simulink model "balance_leg_sl"  (R2022b)
settings: Solver=VariableStepAuto  StartTime=0.0  StopTime=10  RelTol=1e-3
values from neighbouring files (symbols this model uses):
  K = get_K_from_LQR(R_w,R_l,l_l,l_r,l_wl,l_wr,l_bl,l_br,l_c,m_w,m_l,m_b,I_w,I_ll,I_lr,I_b,I_z,g,              R_w_ac,R_l_ac,l_l_ac,l_r_ac,l_wl_ac,l_wr_ac,l_bl_ac,l_br_ac,              l_c_ac,m_w_ac,m_l_ac,m_b_ac,I_w_ac,I_ll_ac,I_lr_ac,I_b_ac,I_z_ac,g_ac,              A,B,lqr_Q,lqr_R)    [HerKules_VOCAL_SJ_LQR_v4_with_data.m]    (also in HerKules_legth_K.m = lqr(A_num, B_num, lqr_Q, lqr_R); get_legth_k.m = lqr(JA,JB,Q,R); lqr_k.m = reshape([mt1,mt2,mt3,mt4,mt5,mt6,mt7,mt8,mt9,mt10,mt11,mt12]; niheK.m = sym('K',[2 6]))
  N = NM + mp*diff(x + L*sin(theta),t,2)    [get_legth_k.m]    (also in niheK.m)
undefined symbols (not defined in the file or in its folder): X, Y, Z
libraries: sm_lib x59, nesl_utility x24, slpidlib x2
(part 1 of 3)
settings Model: Creator=23504  LastModifiedBy=23504

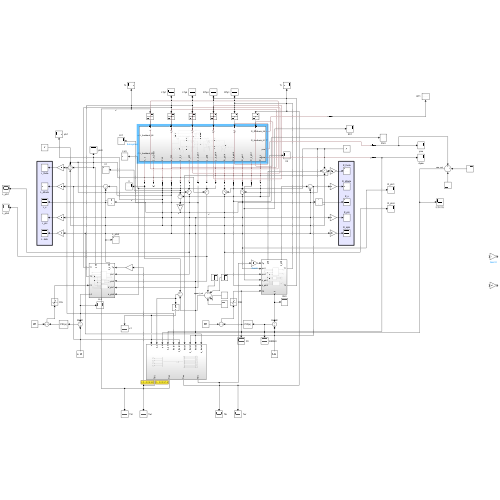
[thumbnail: Simulink's stored preview of the top-level diagram]
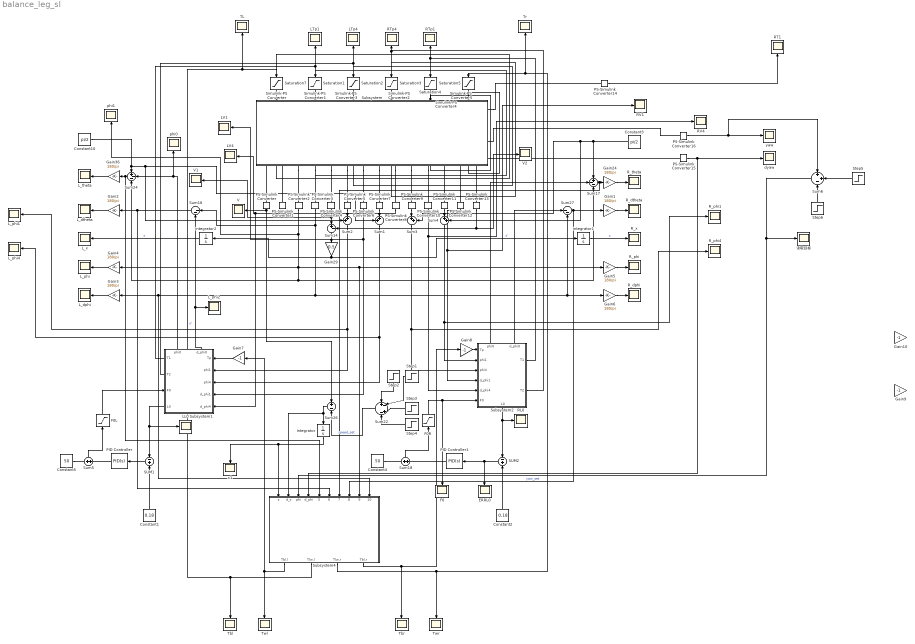
== system balance_leg_sl ==
  Constant1 : Constant  Value=0.18
  Constant10 : Constant  Value=pi/2
  Constant2 : Constant  Value=0.18
  Constant3 : Constant  Value=pi/2
  Constant4 : Constant  Value=50
  Constant5 : Constant  Value=50
  ERRL0 : Scope
  F0 : Scope
  F0L : Saturate  UpperLimit=300  LowerLimit=-300
  F0R : Saturate  UpperLimit=300  LowerLimit=-300
  Gain{1..6,24,36} (8 alike) : Gain  Gain=180/pi
  Gain{7..10} (4 alike) : Gain  Gain=-1
  Gain29 : Gain  Gain=0.5
  Integrator : Integrator
  Integrator1 : Integrator
  Integrator2 : Integrator
  LL0 : Scope
  LTp1 : Scope
  LTp4 : Scope
  LV1 : Scope
  LV4 : Scope
  L_dphi : Scope
  L_dtheta : Scope
  L_phi{,1..2,4} (4 alike) : Scope
  L_theta : Scope
  L_x : Scope
  PID Controller : slpidlib/PID Controller  Controller=PID  Form=Parallel  TimeDomain=Continuous-time  UseExternalTs=off  SampleTime=-1  IntegratorMethod=Forward Euler  FilterMethod=Forward Euler  ControllerParametersSource=internal  P=400  I=100  UseKiTs=off  D=200  N=100  UseFilter=on  TunerSelectOption=Transfer Function Based (PID Tuner App)  InitialConditionSource=internal  InitialConditionForIntegrator=0  InitialConditionForFilter=0  DifferentiatorICPrevScaledInput=0  ExternalReset=none  TrackingMode=off  Kt=1  LimitOutput=off  SatLimitsSource=internal  UpperSaturationLimit=inf  LowerSaturationLimit=-inf  LinearizeAsGain=on  AntiWindupMode=none  Kb=1  LimitIntegrator=off  UpperIntegratorSaturationLimit=inf  LowerIntegratorSaturationLimit=-inf  POutMin=[]  POutMax=[]  IOutMin=[]  IOutMax=[]  DOutMin=[]  DOutMax=[]  NOutMin=[]  NOutMax=[]  SumOutMin=[]  SumOutMax=[]  SaturationOutMin=[]  SaturationOutMax=[]  PParamMin=[]  PParamMax=[]  IParamMin=[]  IParamMax=[]  DParamMin=[]  DParamMax=[]  NParamMin=[]  NParamMax=[]  KbParamMin=[]  KbParamMax=[]  KtParamMin=[]  KtParamMax=[]  KbOutMin=[]  KbOutMax=[]  KtOutMin=[]  KtOutMax=[]  IntegratorOutMin=[]  IntegratorOutMax=[]  FilterOutMin=[]  FilterOutMax=[]  SumI1OutMin=[]  SumI1OutMax=[]  SumI2OutMin=[]  SumI2OutMax=[]  SumI3OutMin=[]  SumI3OutMax=[]  SumI4OutMin=[]  SumI4OutMax=[]  SumDOutMin=[]  SumDOutMax=[]  DifferentiatorOutMin=[]  DifferentiatorOutMax=[]  FilterDiffOutCoefMin=[]  FilterDiffOutCoefMax=[]  ReciprocalOutMin=[]  ReciprocalOutMax=[]  SumDenOutMin=[]  SumDenOutMax=[]  SumNumOutMin=[]  SumNumOutMax=[]  DivideOutMin=[]  DivideOutMax=[]  UdiffTsProdOutMin=[]  UdiffTsProdOutMax=[]  NTsProdOutMin=[]  NTsProdOutMax=[]  UintegralTsProdOutMin=[]  UintegralTsProdOutMax=[]  UngainTsProdOutMin=[]  UngainTsProdOutMax=[]  ClampingZeroOutDataTypeStr=Inherit: Inherit via back propagation  ClampingZeroOutMin=[]  ClampingZeroOutMax=[]  FilterDenConstantOutDataTypeStr=Inherit: Inherit via back propagation  FilterDenConstantOutMin=[]  FilterDenConstantOutMax=[]  PCopyOutDataTypeStr=Inherit: Inherit via back propagation  PCopyOutMin=[]  PCopyOutMax=[]  NCopyOutDataTypeStr=Inherit: Inherit via back propagation  NCopyOutMin=[]  NCopyOutMax=[]  IntegratorContinuousStateAttributes=''  IntegratorStateMustResolveToSignalObject=off  IntegratorRTWStateStorageClass=Auto  FilterContinuousStateAttributes=''  FilterStateMustResolveToSignalObject=off  FilterRTWStateStorageClass=Auto  ParallelPVariant=InternalParameters  IdealPVariant=Disabled  IVariant=InternalParameters  DVariant=InternalParameters  IntegratorVariant=Continuous  SatVariant=Disabled  AWVariant=Passthrough  PCopyVariant=Disabled  TRVariant=Disabled  FdbkBlocksVariant=Forward  IdealPFdbkVariant=Disabled  SatFdbkVariant=Disabled  DerivativeFilterVariant=ContFilter  NVariant=InternalParameters  NCopyVariant=Disabled  FilterICVariant=InternalICsFilter  IntegratorICVariant=InternalICs  ExternalResetVariant=Disabled  TRSumVariant=Passthrough  SumFdbkVariant=Disabled  SumVariant=Sum_PID  TsampFilterVariant=InternalTs  TsampNgainVariant=Passthrough  TsampIntegralVariant=Passthrough  ExternalSaturationOutDataTypeStr=Inherit: Same as second input
  PID Controller1 : slpidlib/PID Controller  Controller=PID  Form=Parallel  TimeDomain=Continuous-time  UseExternalTs=off  SampleTime=-1  IntegratorMethod=Forward Euler  FilterMethod=Forward Euler  ControllerParametersSource=internal  P=400  I=100  UseKiTs=off  D=200  N=100  UseFilter=on  TunerSelectOption=Transfer Function Based (PID Tuner App)  InitialConditionSource=internal  InitialConditionForIntegrator=0  InitialConditionForFilter=0  DifferentiatorICPrevScaledInput=0  ExternalReset=none  TrackingMode=off  Kt=1  LimitOutput=off  SatLimitsSource=internal  UpperSaturationLimit=inf  LowerSaturationLimit=-inf  LinearizeAsGain=on  AntiWindupMode=none  Kb=1  LimitIntegrator=off  UpperIntegratorSaturationLimit=inf  LowerIntegratorSaturationLimit=-inf  POutMin=[]  POutMax=[]  IOutMin=[]  IOutMax=[]  DOutMin=[]  DOutMax=[]  NOutMin=[]  NOutMax=[]  SumOutMin=[]  SumOutMax=[]  SaturationOutMin=[]  SaturationOutMax=[]  PParamMin=[]  PParamMax=[]  IParamMin=[]  IParamMax=[]  DParamMin=[]  DParamMax=[]  NParamMin=[]  NParamMax=[]  KbParamMin=[]  KbParamMax=[]  KtParamMin=[]  KtParamMax=[]  KbOutMin=[]  KbOutMax=[]  KtOutMin=[]  KtOutMax=[]  IntegratorOutMin=[]  IntegratorOutMax=[]  FilterOutMin=[]  FilterOutMax=[]  SumI1OutMin=[]  SumI1OutMax=[]  SumI2OutMin=[]  SumI2OutMax=[]  SumI3OutMin=[]  SumI3OutMax=[]  SumI4OutMin=[]  SumI4OutMax=[]  SumDOutMin=[]  SumDOutMax=[]  DifferentiatorOutMin=[]  DifferentiatorOutMax=[]  FilterDiffOutCoefMin=[]  FilterDiffOutCoefMax=[]  ReciprocalOutMin=[]  ReciprocalOutMax=[]  SumDenOutMin=[]  SumDenOutMax=[]  SumNumOutMin=[]  SumNumOutMax=[]  DivideOutMin=[]  DivideOutMax=[]  UdiffTsProdOutMin=[]  UdiffTsProdOutMax=[]  NTsProdOutMin=[]  NTsProdOutMax=[]  UintegralTsProdOutMin=[]  UintegralTsProdOutMax=[]  UngainTsProdOutMin=[]  UngainTsProdOutMax=[]  ClampingZeroOutDataTypeStr=Inherit: Inherit via back propagation  ClampingZeroOutMin=[]  ClampingZeroOutMax=[]  FilterDenConstantOutDataTypeStr=Inherit: Inherit via back propagation  FilterDenConstantOutMin=[]  FilterDenConstantOutMax=[]  PCopyOutDataTypeStr=Inherit: Inherit via back propagation  PCopyOutMin=[]  PCopyOutMax=[]  NCopyOutDataTypeStr=Inherit: Inherit via back propagation  NCopyOutMin=[]  NCopyOutMax=[]  IntegratorContinuousStateAttributes=''  IntegratorStateMustResolveToSignalObject=off  IntegratorRTWStateStorageClass=Auto  FilterContinuousStateAttributes=''  FilterStateMustResolveToSignalObject=off  FilterRTWStateStorageClass=Auto  ParallelPVariant=InternalParameters  IdealPVariant=Disabled  IVariant=InternalParameters  DVariant=InternalParameters  IntegratorVariant=Continuous  SatVariant=Disabled  AWVariant=Passthrough  PCopyVariant=Disabled  TRVariant=Disabled  FdbkBlocksVariant=Forward  IdealPFdbkVariant=Disabled  SatFdbkVariant=Disabled  DerivativeFilterVariant=ContFilter  NVariant=InternalParameters  NCopyVariant=Disabled  FilterICVariant=InternalICsFilter  IntegratorICVariant=InternalICs  ExternalResetVariant=Disabled  TRSumVariant=Passthrough  SumFdbkVariant=Disabled  SumVariant=Sum_PID  TsampFilterVariant=InternalTs  TsampNgainVariant=Passthrough  TsampIntegralVariant=Passthrough  ExternalSaturationOutDataTypeStr=Inherit: Same as second input
  PS-Simulink Converter{,1..16} (17 alike) : nesl_utility/PS-Simulink Converter  PhysicalDomain=network_engine_domain  SubClassName=ps_output  LeftPortType=input  RightPortType=output  PseudoPeriodic=off  Frequencies=[]  VectorFormat=inherit  Unit=inherit  AffineConversion=off
  RL0 : Scope
  RT1 : Scope
  RTp1 : Scope
  RTp4 : Scope
  RV1 : Scope
  RV4 : Scope
  R_dphi : Scope
  R_dtheta : Scope
  R_phi : Scope
  R_phi1 : Scope
  R_phi4 : Scope
  R_theta : Scope
  R_x : Scope
  SUM1 : Sum  Inputs=-|+
  SUM2 : Sum  Inputs=-|+
  Saturation{1..4} (4 alike) : Saturate  UpperLimit=100  LowerLimit=-100
  Saturation5 : Saturate  UpperLimit=9  LowerLimit=-9
  Saturation7 : Saturate  UpperLimit=9  LowerLimit=-9
  Simulink-PS Converter{,1..5} (6 alike) : nesl_utility/Simulink-PS Converter  PhysicalDomain=network_engine_domain  SubClassName=ps_input  LeftPortType=input  RightPortType=output  PseudoPeriodic=off  Frequencies=[]  NoiseDistribution=none  NoiseParameters=[]  Unit=1  AffineConversion=off  FilteringAndDerivatives=provide  SimscapeFilterOrder=1  InputFilterTimeConstant=0.001  UdotUserProvided=0
  Step1 : Step  Time=3  After=1.5  SampleTime=0
  Step2 : Step  Time=0.8  After=1.5  SampleTime=0
  Step3 : Step  Time=5  After=-1.5  SampleTime=0
  Step4 : Step  Time=7.2  After=-1.5  SampleTime=0
  Step5 : Step  Time=7  After=0.5  SampleTime=0
  Step6 : Step  Time=3  After=0.5  SampleTime=0
  Subsystem : Subsystem
      settings: PortSchema="{\"entries\":[{\"content\":{\"sides\":[{\"content\":{\"connectorIds\":[\"LConn1\",\"LConn2\",\"LConn3\",\"LConn4\",\"LConn5\",\"LConn6\"]},\"type\":\"ConnectorPlacement.EquallySpacedRectSide\",\"uuid\":\"cf554540-2f59-4125-b9e8-e473df85a330\"},{\"content\":{\"connectorIds\":[\"RConn1\",\"RConn2\",\"RConn3\",\"RConn4\",\"RConn5\",\"RConn6\",\"RConn7\",\"RConn8\",\"RConn9\",\"RConn10\",\"RConn11\",\"RConn12\",\"RConn13\",\"RConn14\"],\"side\":\"RIGHT\"},\"type\":\"ConnectorPlacement.EquallySpacedRectSide\",\"uuid\":\"e23304d1-39ba-424b-95c6-dea28be1cd8e\"},{\"content\":{\"connectorIds\":[\"LConn7\",\"LConn8\"],\"side\":\"TOP\"},\"type\":\"ConnectorPlacement.EquallySpacedRectSide\",\"uuid\":\"7a5e8007-1d8b-4e1b-a20d-f8b506f10684\"},{\"content\":{\"connectorIds\":[\"RConn15\",\"RConn16\",\"RConn17\",\"RConn18\"],\"side\":\"BOTTOM\"},\"type\":\"ConnectorPlacement.EquallySpacedRectSide\",\"uuid\":\"9af58ce4-847d-4aa1-92fa-5098b5cad22e\"}]},\"type\":\"ConnectorPlacement.EquallySpacedConnector\",\"uuid\":\"bed63bae-ae77-4c2c-be48-a3ad435d1975\"}],\"packageUris\":[\"http://schema.mathworks.com/mf0/Connector/R2020b\"],\"version\":\"1.0\"}"
  Subsystem1 : Subsystem
      settings: PortSchema="{\"entries\":[{\"content\":{\"sides\":[{\"content\":{\"connectorIds\":[\"In1\",\"In2\",\"In3\",\"In4\",\"In5\"]},\"type\":\"ConnectorPlacement.EquallySpacedRectSide\",\"uuid\":\"bfceb98f-1d5a-45d0-a562-d65d98f91de3\"},{\"content\":{\"connectorIds\":[\"Out1\",\"Out2\",\"In6\",\"Out3\"],\"side\":\"RIGHT\"},\"type\":\"ConnectorPlacement.EquallySpacedRectSide\",\"uuid\":\"b8c5e340-7cee-4107-8ea2-3c9753bc0d7d\"},{\"content\":{\"connectorIds\":[\"Out4\",\"Out5\"],\"side\":\"TOP\"},\"type\":\"ConnectorPlacement.EquallySpacedRectSide\",\"uuid\":\"ffdc1c07-0318-4ba0-a86f-ac17560f0ac1\"}]},\"type\":\"ConnectorPlacement.EquallySpacedConnector\",\"uuid\":\"09be8c59-74e0-434b-a6e6-bc357885ae04\"}],\"packageUris\":[\"http://schema.mathworks.com/mf0/Connector/R2020b\"],\"version\":\"1.0\"}"
  Subsystem2 : Subsystem
      settings: PortSchema="{\"entries\":[{\"content\":{\"sides\":[{\"content\":{\"connectorIds\":[\"In1\",\"In2\",\"In3\",\"In4\",\"In5\",\"In6\"]},\"type\":\"ConnectorPlacement.EquallySpacedRectSide\",\"uuid\":\"bfceb98f-1d5a-45d0-a562-d65d98f91de3\"},{\"content\":{\"connectorIds\":[\"Out1\",\"Out2\"],\"side\":\"RIGHT\"},\"type\":\"ConnectorPlacement.EquallySpacedRectSide\",\"uuid\":\"b8c5e340-7cee-4107-8ea2-3c9753bc0d7d\"},{\"content\":{\"connectorIds\":[\"Out4\",\"Out5\"],\"side\":\"TOP\"},\"type\":\"ConnectorPlacement.EquallySpacedRectSide\",\"uuid\":\"ffdc1c07-0318-4ba0-a86f-ac17560f0ac1\"},{\"content\":{\"connectorIds\":[\"Out3\"],\"side\":\"BOTTOM\"},\"type\":\"ConnectorPlacement.EquallySpacedRectSide\",\"uuid\":\"f7d6fcc6-80be-453b-bdb0-f278a7db9a79\"}]},\"type\":\"ConnectorPlacement.EquallySpacedConnector\",\"uuid\":\"09be8c59-74e0-434b-a6e6-bc357885ae04\"}],\"packageUris\":[\"http://schema.mathworks.com/mf0/Connector/R2020b\"],\"version\":\"1.0\"}"
  Subsystem4 : Subsystem
  Sum1 : Sum  Inputs=++|
  Sum14 : Sum  Inputs=|+-
  Sum16 : Sum  Inputs=|--
  Sum17 : Sum  Inputs=+--
  Sum18 : Sum  Inputs=+|+
  Sum2 : Sum  Inputs=++|
  Sum22 : Sum  Inputs=+-|+-
  Sum24 : Sum  Inputs=+--
  Sum26 : Sum  Inputs=+-
  Sum27 : Sum  Inputs=|--
  Sum3 : Sum  Inputs=|++
  Sum4 : Sum  Inputs=|++
  Sum5 : Sum  Inputs=+|+
  Sum6 : Sum  Inputs=++-
  TL : Scope
  Tbl : Scope
  Tbr : Scope
  Tr : Scope
  Twl : Scope
  Twr : Scope
  V : Scope
  V1 : Scope
  V2 : Scope
  dyaw : Scope
  phi0 : Scope
  phi1 : Scope
  x1 : Scope
  yaw : Scope
  读取目标 : Scope
  wires:
  PS-Simulink Converter11/1 -> Sum4/1
  Constant2/1 -> SUM2/2
  PS-Simulink Converter2/1 -> phi1/1, Subsystem4/9(thetab), Gain5/1, Gain4/1, Sum24/3, Sum17/3
  PS-Simulink Converter8/1 -> LV4/1, Subsystem1/5(d_phi4)
  Step2/1 -> Sum22/1
  SUM2/1 -> ERRL0/1, PID Controller1/1
  Gain24/1 -> R_theta/1
  Subsystem1/1(T1) -> Saturation1/1, LTp1/1
  PS-Simulink Converter14/1 -> RT1/1
  Constant4/1 -> Sum18/1
  Gain4/1 -> L_phi/1
  Gain3/1 -> L_dphi/1
  Subsystem1/4(d_phi0) -> Sum16/2, L_phi2/1
  Step3/1 -> Sum22/3
  PS-Simulink Converter9/1 -> Sum3/1
  Sum16/1 -> Gain2/1, Subsystem4/6(d_thetall)
  Step4/1 -> Sum22/4
  Saturation1/1 -> Simulink-PS Converter1/1
  Sum18/1 -> F0R/1
  Subsystem2/4(phi0) -> Sum17/2
  PID Controller/1 -> Sum5/2
  PS-Simulink Converter6/1 -> LV1/1, Subsystem1/4(d_phi1)
  Sum5/1 -> F0L/1
  Sum22/1 -> Sum26/2  "speed_set"
  Constant5/1 -> Sum5/1
  Subsystem2/2(T2) -> Saturation3/1, RTp4/1
  PS-Simulink Converter5/1 -> Sum2/2
  SUM1/1 -> PID Controller/1
  Sum2/1 -> L_phi1/1, Subsystem1/2(phi1)
  PID Controller1/1 -> Sum18/2
  PS-Simulink Converter/1 -> V/1, Sum26/1
  PS-Simulink Converter12/1 -> RV1/1, Subsystem2/4(d_phi1)
  PS-Simulink Converter10/1 -> RV4/1, Subsystem2/5(d_phi4)
  Gain5/1 -> R_phi/1
  PS-Simulink Converter7/1 -> Sum1/2
  Subsystem2/5(d_phi0) -> Sum27/1
  PS-Simulink Converter3/1 -> Sum16/1, Sum27/2, Gain6/1, Gain3/1, Subsystem4/10(d_thetab)
  Gain6/1 -> R_dphi/1
  Gain2/1 -> L_dtheta/1
  Sum3/1 -> R_phi4/1, Subsystem2/3(phi4)
  Sum4/1 -> R_phi1/1, Subsystem2/2(phi1)
  Sum1/1 -> L_phi4/1, Subsystem1/3(phi4)
  Sum26/1 -> Subsystem4/2(d_s), Integrator/1
  Integrator/1 -> x1/1, Subsystem4/1(s)
  Gain36/1 -> L_theta/1
  Step1/1 -> Sum22/2
  Subsystem1/5(phi0) -> phi0/1, Sum24/2
  Subsystem2/3(L0) -> SUM2/1, RL0/1
  Integrator1/1 -> R_x/1  "x"
  Sum24/1 -> Subsystem4/5(thetall), Gain36/1
  Sum17/1 -> Subsystem4/7(thetalr), Gain24/1
  Sum27/1 -> Subsystem4/8(d_thetalr), Gain1/1
  Constant1/1 -> SUM1/2
  Constant3/1 -> Sum4/2, Sum3/2, Sum17/1
  Subsystem2/1(T1) -> RTp1/1, Saturation4/1
  Subsystem1/3(L0) -> LL0/1, SUM1/1
  PS-Simulink Converter4/1 -> V1/1, Sum14/1
  Saturation2/1 -> Simulink-PS Converter3/1
  Sum14/1 -> Gain29/1
  Constant10/1 -> Sum2/1, Sum1/1, Sum24/1
  Saturation7/1 -> Simulink-PS Converter/1
  PS-Simulink Converter13/1 -> V2/1, Sum14/2
  F0L/1 -> Subsystem1/6(F0)
  Saturation3/1 -> Simulink-PS Converter2/1
  Saturation5/1 -> Simulink-PS Converter5/1
  Gain29/1 -> Integrator1/1, Integrator2/1  "x'"
  Gain1/1 -> R_dtheta/1
  Integrator2/1 -> L_x/1  "x"
  Saturation4/1 -> Simulink-PS Converter4/1
  F0R/1 -> Subsystem2/6(F0), F0/1
  Subsystem1/2(T2) -> LTp4/1, Saturation2/1
  Subsystem4/2(Tlw,l) -> Tbl/1, TL/1, Saturation7/1  "x'"
  Subsystem4/1(Tbl,l) -> Gain7/1, Twl/1
  Subsystem4/3(Tlw,r) -> Twr/1, Saturation5/1, Tr/1
  Subsystem4/4(Tbl,r) -> Gain8/1, Tbr/1
  PS-Simulink Converter16/1 -> Sum6/1, yaw/1
  PS-Simulink Converter15/1 -> dyaw/1, Subsystem4/4(d_phi)
  Gain7/1 -> Subsystem1/1(Tp)
  Gain8/1 -> Subsystem2/1(Tp)
  Step6/1 -> Sum6/3
  Step5/1 -> Sum6/2
  Sum6/1 -> 读取目标/1, Subsystem4/3(phi)  "yaw_set"
  connections:
  Subsystem/RConn15 -- PS-Simulink Converter14/LConn1
  Subsystem/RConn8 -- PS-Simulink Converter7/LConn1
  Subsystem/RConn7 -- PS-Simulink Converter6/LConn1
  Subsystem/RConn9 -- PS-Simulink Converter8/LConn1
  Subsystem/RConn11 -- PS-Simulink Converter10/LConn1
  Subsystem/RConn6 -- PS-Simulink Converter5/LConn1
  Subsystem/LConn5 -- Simulink-PS Converter4/RConn1
  Simulink-PS Converter2/RConn1 -- Subsystem/LConn4
  Subsystem/RConn3 -- PS-Simulink Converter2/LConn1
  Simulink-PS Converter3/RConn1 -- Subsystem/LConn3
  Subsystem/RConn12 -- PS-Simulink Converter11/LConn1
  Subsystem/RConn5 -- PS-Simulink Converter4/LConn1
  Simulink-PS Converter/RConn1 -- Subsystem/LConn1
  PS-Simulink Converter1/LConn1 -- Subsystem/RConn2
  Subsystem/RConn10 -- PS-Simulink Converter9/LConn1
  Subsystem/RConn13 -- PS-Simulink Converter12/LConn1
  Subsystem/RConn4 -- PS-Simulink Converter3/LConn1
  Subsystem/RConn14 -- PS-Simulink Converter13/LConn1
  PS-Simulink Converter/LConn1 -- Subsystem/RConn1
  Simulink-PS Converter1/RConn1 -- Subsystem/LConn2
  Subsystem/LConn6 -- Simulink-PS Converter5/RConn1
  Subsystem/RConn17 -- PS-Simulink Converter16/LConn1
  Subsystem/RConn18 -- PS-Simulink Converter15/LConn1
